simulink model "DFII"  (R2014a)
settings: Solver=FixedStepDiscrete  StartTime=0.0  StopTime=1  FixedStep=1e-2  RelTol=1e-3
values from neighbouring files (symbols this model uses):
  a = sos(:, 4:6)    [LowpassFilter.m]
  b = sos(:, 1:3)    [LowpassFilter.m]
settings Model: Creator=Vincent  LastModifiedBy=Vincent

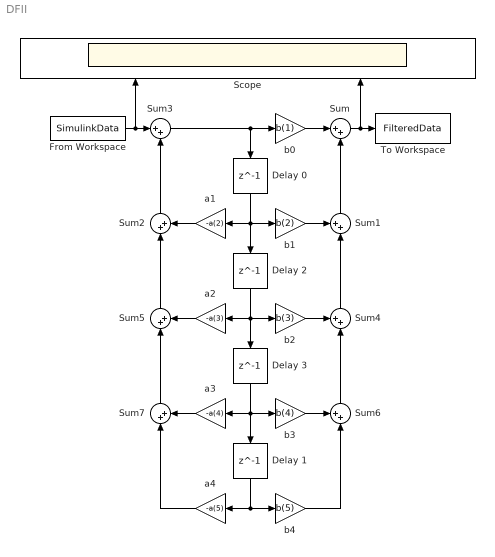
== system DFII ==
  Delay {0..3} (4 alike) : Delay  DelayLength=1  InitialCondition=0
  From Workspace : FromWorkspace  VariableName=SimulinkData  SampleTime=0
  Scope : Scope  NumInputPorts=2
      settings: YMin=-5~-5  YMax=5~5
  Sum{,2..3,5,7} (5 alike) : Sum  Inputs=|++
  Sum1 : Sum  Inputs=++|
  Sum4 : Sum  Inputs=++|
  Sum6 : Sum  Inputs=++|
  To Workspace : ToWorkspace  VariableName=FilteredData  SaveFormat=Structure With Time  SampleTime=-1
  a1 : Gain  Gain=-a(2)
  a2 : Gain  Gain=-a(3)
  a3 : Gain  Gain=-a(4)
  a4 : Gain  Gain=-a(5)
  b0 : Gain  Gain=b(1)
  b1 : Gain  Gain=b(2)
  b2 : Gain  Gain=b(3)
  b3 : Gain  Gain=b(4)
  b4 : Gain  Gain=b(5)
  wires:
  b0/1 -> Sum/1
  Sum/1 -> Scope/2, To Workspace/1
  b1/1 -> Sum1/1
  Delay 0/1 -> Delay 2/1, a1/1, b1/1
  a1/1 -> Sum2/2
  Sum2/1 -> Sum3/2
  From Workspace/1 -> Scope/1, Sum3/1
  Sum3/1 -> b0/1, Delay 0/1
  Sum1/1 -> Sum/2
  b2/1 -> Sum4/1
  Delay 2/1 -> Delay 3/1, a2/1, b2/1
  a2/1 -> Sum5/2
  Sum5/1 -> Sum2/1
  Sum4/1 -> Sum1/2
  Delay 1/1 -> a4/1, b4/1
  a4/1 -> Sum7/1
  b4/1 -> Sum6/2
  b3/1 -> Sum6/1
  Delay 3/1 -> Delay 1/1, a3/1, b3/1
  a3/1 -> Sum7/2
  Sum7/1 -> Sum5/1
  Sum6/1 -> Sum4/2
